simulink model "Dcmotor"  (R2022a)
settings: Solver=VariableStepAuto  StartTime=0.0  StopTime=10.0  RelTol=1e-3
settings Model: Creator=asopi  LastModifiedBy=asopi

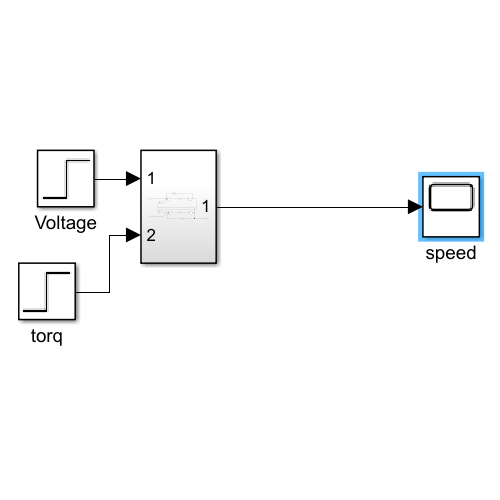
[thumbnail: Simulink's stored preview of the top-level diagram]
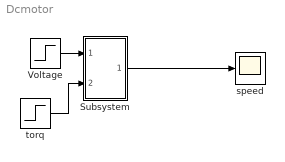
== system Dcmotor ==
  Subsystem : Subsystem
  Voltage : Step  After=2  SampleTime=0
  speed : Scope
  torq : Step  SampleTime=0
  wires:
  Voltage/1 -> Subsystem/1(In1)
  Subsystem/1(Out1) -> speed/1
  torq/1 -> Subsystem/2(In2)

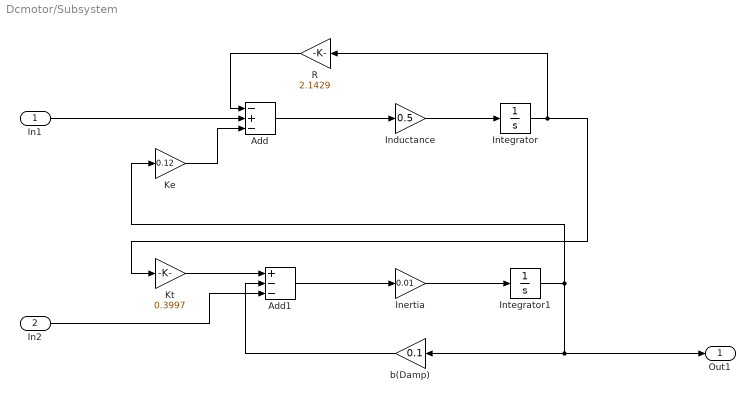
== system Dcmotor/Subsystem ==
  In1 : Inport
  In2 : Inport  Port=2
  Add : Sum  Inputs=-+-
  Add1 : Sum  Inputs=+--
  Inductance : Gain  Gain=0.5
  Inertia : Gain  Gain=0.01
  Integrator : Integrator
  Integrator1 : Integrator
  Ke : Gain  Gain=0.12
  Kt : Gain  Gain=0.3997
  R : Gain  Gain=2.1429
  b(Damp) : Gain  Gain=0.1
  Out1 : Outport
  wires:
  Kt/1 -> Add1/1
  Ke/1 -> Add/3
  R/1 -> Add/1
  Add/1 -> Inductance/1
  Integrator1/1 -> Ke/1, Out1/1, b(Damp)/1
  Inductance/1 -> Integrator/1
  Add1/1 -> Inertia/1
  b(Damp)/1 -> Add1/2
  Inertia/1 -> Integrator1/1
  Integrator/1 -> R/1, Kt/1
  In1/1 -> Add/2
  In2/1 -> Add1/3
